simulink model "RL_Model"  (R2021a)
settings: Solver=ode45  StartTime=0.0  StopTime=100  RelTol=1e-3  EnableMultiTasking=on
undefined symbols (not defined in the file): DiscIntNeverNeededParam, Ts
libraries: simulink x3, rllib x1
settings Model: Creator=The MathWorks, Inc.  LastModifiedBy=Daniel A. Udekwe
settings SolverCC: AlgebraicLoopSolver=TrustRegion
settings DataIOCC: LimitDataPoints=on  SaveFormat=Array  ReturnWorkspaceOutputs=off  SignalLoggingName=logsOut
settings OptimizationCC: ExpressionDepthLimit=2147483647  InitFltsAndDblsToZero=on  LifeSpan=inf
settings DebuggingCC: SaveWithParameterizedLinksMsg=none  UnderspecifiedInitializationDetection=Classic  MergeDetectMultiDrivingBlocksExec=none  SignalResolutionControl=TryResolveAllWithWarning  MultiTaskDSMMsg=warning  FcnCallInpInsideContextMsg=warning  AllowSymbolicDim=off  StateNameClashWarn=warning  SFUnexpectedBacktrackingDiag=warning  SFNoUnconditionalDefaultTransitionDiag=warning  SFExecutionAtInitializationDiag=none  SFMachineParentedDataDiag=warning  ArithmeticOperatorsInVariantConditions=warning
settings HardwareCC: ProdBitPerPointer=32  ProdBitPerSizeT=32  ProdBitPerPtrDiffT=32  ProdLargestAtomicFloat=None  ProdIntDivRoundTo=Undefined  ProdEndianess=Unspecified  ProdWordSize=32  ProdHWDeviceType=Specified
settings ModelReferenceCC: PropagateSignalLabelsOutOfModel=off
settings SFSimCC: SimUseLocalCustomCode=off  CustomCodeUndefinedFunction=UseInterfaceOnly
settings RTWCC: RTWUseLocalCustomCode=off
settings CodeAppCC: StateflowObjectComments=on
settings GRTTargetCC: TargetFcnLib=ansi_tfl_tmw.mat  TargetLangStandard=C89/C90 (ANSI)  CombineOutputUpdateFcns=off  GRTInterface=on
settings ConfigComp: CovMetricSettings=dw  CovSaveCumulativeToWorkspaceVar=on  CovSaveSingleToWorkspaceVar=on  CovExternalEMLEnable=off

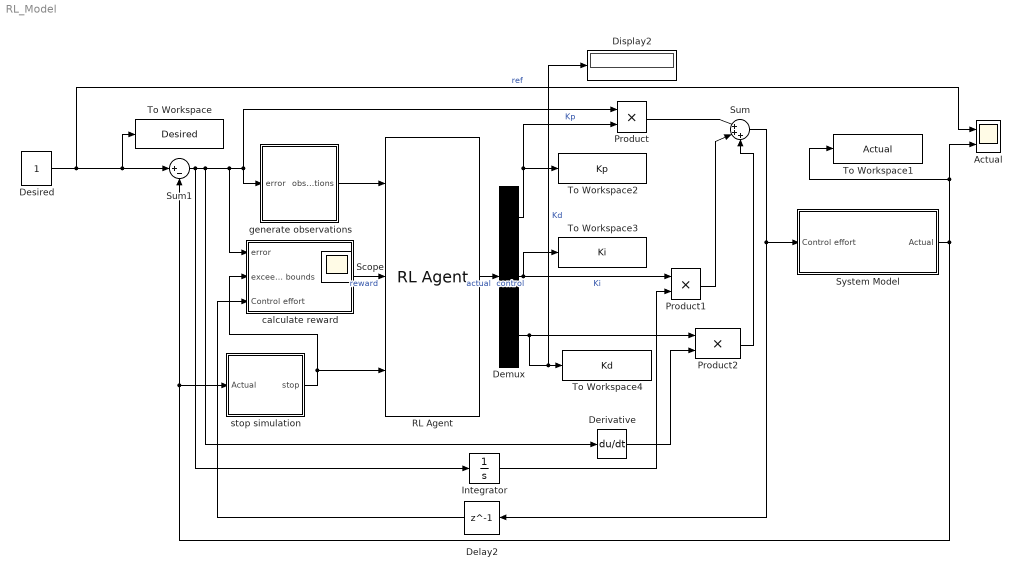
== system RL_Model ==
  Actual : Scope  NumInputPorts=2
  Delay2 : Delay  DelayLength=1
  Demux : Demux  Outputs=3
  Derivative : Derivative  CoefficientInTFapproximation=0
  Desired : Constant
  Display2 : Display
  Integrator : Integrator
  Product : Product
  Product1 : Product
  Product2 : Product
  RL Agent : rllib/RL Agent  Agent=agent  ExternalActionAsInput=off  ProvideCumRwd=off  TreatAsDirectFeedthrough=on
  Sum : Sum  Inputs=|+++
  Sum1 : Sum  Inputs=|+-  SaturateOnIntegerOverflow=on
  System Model : Subsystem
  To Workspace : ToWorkspace  VariableName=Desired  SampleTime=-1
  To Workspace1 : ToWorkspace  VariableName=Actual  SampleTime=-1
  To Workspace2 : ToWorkspace  VariableName=Kp  SaveFormat=Structure With Time  SampleTime=-1
  To Workspace3 : ToWorkspace  VariableName=Ki  SaveFormat=Structure With Time  SampleTime=-1
  To Workspace4 : ToWorkspace  VariableName=Kd  SaveFormat=Structure With Time  SampleTime=-1
  calculate reward : Subsystem
  generate observations : Subsystem
  stop simulation : Subsystem
  Scope : Scope
  wires:
  Sum1/1 -> generate observations/1(error), Product/1, calculate reward/1(error), Derivative/1, Integrator/1
  stop simulation/1(stop) -> RL Agent/3, calculate reward/2(exceeds bounds)
  calculate reward/1(reward) -> RL Agent/2  "reward"
  generate observations/1(observations) -> RL Agent/1
  System Model/1(Actual) -> Actual/2, To Workspace1/1, stop simulation/1(Actual), Sum1/2
  RL Agent/1 -> Demux/1  "actual  control"
  Demux/1 -> Product/2, To Workspace2/1  "Kp"
  Product/1 -> Sum/1
  Integrator/1 -> Product1/2
  Product1/1 -> Sum/2
  Demux/2 -> To Workspace3/1, Product1/1  "Ki"
  Demux/3 -> Product2/1, Display2/1, To Workspace4/1  "Kd"
  Derivative/1 -> Product2/2
  Product2/1 -> Sum/3
  Desired/1 -> Actual/1, To Workspace/1, Sum1/1  "ref"
  Sum/1 -> Delay2/1, System Model/1(Control effort)
  Delay2/1 -> calculate reward/3(Control effort)

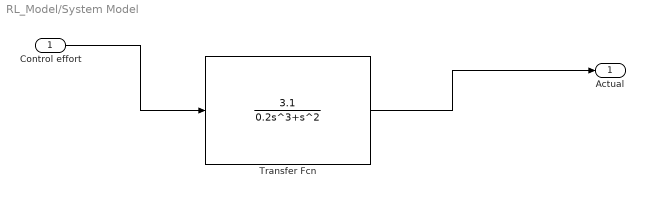
== system RL_Model/System Model ==
  Control effort : Inport
  Transfer Fcn : TransferFcn  Numerator=[3.1]  Denominator=[0.2 1 0 0]
  Actual : Outport  VectorParamsAs1DForOutWhenUnconnected=off
  wires:
  Transfer Fcn/1 -> Actual/1
  Control effort/1 -> Transfer Fcn/1

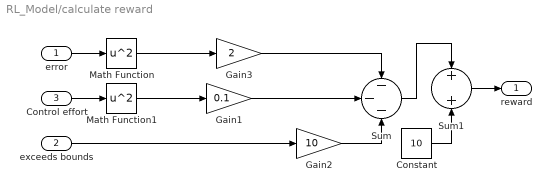
== system RL_Model/calculate reward ==
  error : Inport
  exceeds bounds : Inport  Port=2
  Control effort : Inport  Port=3
  Constant : Constant  Value=10
  Gain1 : Gain  Gain=0.1
  Gain2 : Gain  Gain=10
  Gain3 : Gain  Gain=2
  Math Function : Math  Operator=square  SaturateOnIntegerOverflow=on
  Math Function1 : Math  Operator=square  SaturateOnIntegerOverflow=on
  Sum : Sum  Inputs=---  OutDataTypeStr=double
  Sum1 : Sum  OutDataTypeStr=double
  reward : Outport  VectorParamsAs1DForOutWhenUnconnected=off
  wires:
  exceeds bounds/1 -> Gain2/1
  error/1 -> Math Function/1
  Math Function/1 -> Gain3/1
  Gain3/1 -> Sum/1
  Sum/1 -> Sum1/1
  Constant/1 -> Sum1/2
  Sum1/1 -> reward/1
  Math Function1/1 -> Gain1/1
  Gain2/1 -> Sum/3
  Control effort/1 -> Math Function1/1
  Gain1/1 -> Sum/2

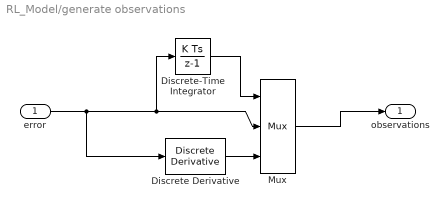
== system RL_Model/generate observations ==
  error : Inport
  Discrete Derivative : simulink/Discrete/Discrete Derivative  gainval=1.0  ICPrevScaledInput=0.0  OutMin=[]  OutMax=[]  OutDataType=fixdt(1, 16)  OutScaling=2^-10  DoSatur=off
  Discrete-Time Integrator : DiscreteIntegrator  SampleTime=Ts  ICPrevOutput=DiscIntNeverNeededParam  ICPrevScaledInput=DiscIntNeverNeededParam
  Mux : Mux  Inputs=3
  observations : Outport  VectorParamsAs1DForOutWhenUnconnected=off
  wires:
  Discrete-Time Integrator/1 -> Mux/1
  error/1 -> Discrete Derivative/1, Discrete-Time Integrator/1, Mux/2
  Mux/1 -> observations/1
  Discrete Derivative/1 -> Mux/3

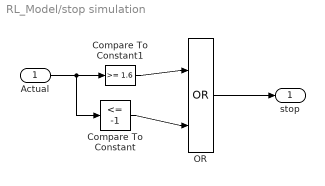
== system RL_Model/stop simulation ==
  Actual : Inport
  Compare To Constant : simulink/Logic and Bit Operations/Compare To Constant  relop=<=  const=-1  OutDataTypeStr=boolean
  Compare To Constant1 : simulink/Logic and Bit Operations/Compare To Constant  relop=>=  const=1.6  OutDataTypeStr=boolean
  OR : Logic  Operator=OR  IconShape=distinctive  AllPortsSameDT=off  OutDataTypeStr=boolean
  stop : Outport  VectorParamsAs1DForOutWhenUnconnected=off
  wires:
  Actual/1 -> Compare To Constant/1, Compare To Constant1/1
  Compare To Constant/1 -> OR/2
  Compare To Constant1/1 -> OR/1
  OR/1 -> stop/1
